simulink model "CRIT4INDIFullLoop"  (R2019b)
settings: Solver=VariableStepAuto  StartTime=0.0  StopTime=50  RelTol=1e-3
values from neighbouring files (symbols this model uses):
  Ahg2 = blkdiag(Ahg2, Ahcg)    [HinFSynINDIFullLoop.m]
  Ahs3 = blkdiag(Ahs3, Ahcs)    [HinFSynINDIFullLoop.m]
  Ahs7 = blkdiag(Ahs7, Ahcs)    [HinFSynINDIFullLoop.m]
  Amc = d2c(Amd,'tustin')    [HinFSynINDIFullLoop.m]
  Asc = d2c(Asd,'tustin')    [HinFSynINDIFullLoop.m]
  Bhg2 = blkdiag(Bhg2, Bhcg)    [HinFSynINDIFullLoop.m]
  Bhs3 = blkdiag(Bhs3, Bhcs)    [HinFSynINDIFullLoop.m]
  Bhs7 = blkdiag(Bhs7, Bhcs)    [HinFSynINDIFullLoop.m]
  Chg2 = blkdiag(Chg2, Chcg)    [HinFSynINDIFullLoop.m]
  Chs3 = blkdiag(Chs3, Chcs)    [HinFSynINDIFullLoop.m]
  Chs7 = blkdiag(Chs7, Chcs)    [HinFSynINDIFullLoop.m]
  Dhg2 = blkdiag(Dhg2, Dhcg)    [HinFSynINDIFullLoop.m]
  Dhs3 = blkdiag(Dhs3, Dhcs)    [HinFSynINDIFullLoop.m]
  Dhs7 = blkdiag(Dhs7, Dhcs)    [HinFSynINDIFullLoop.m]
  Gs = [-10.67  10.67  0     0     0     0 0 ... (first row only)    [HinFSynINDIFullLoop.m]
  Gs_inv = pinv(Gs)    [HinFSynINDIFullLoop.m]
  Gs_thrust = [0 0 0 0 0 0 0 ... (first row only)    [HinFSynINDIFullLoop.m]
  Kdg = diag([2.0; 1.8])    [HinFSynINDIFullLoop.m]
  Kds = [10; 18; 18]    [HinFSynINDIFullLoop.m]
  Kpg = blkdiag(Kposx.D,Kposz.D)    [HinFSynINDIFullLoop.m]
  Kps = [4.1089; 4.7304; 7.36]    [HinFSynINDIFullLoop.m]
settings Model: Creator=AutomZ2-RG02A02  LastModifiedBy=demouran
settings DebuggingCC: SFMachineParentedDataDiag=error

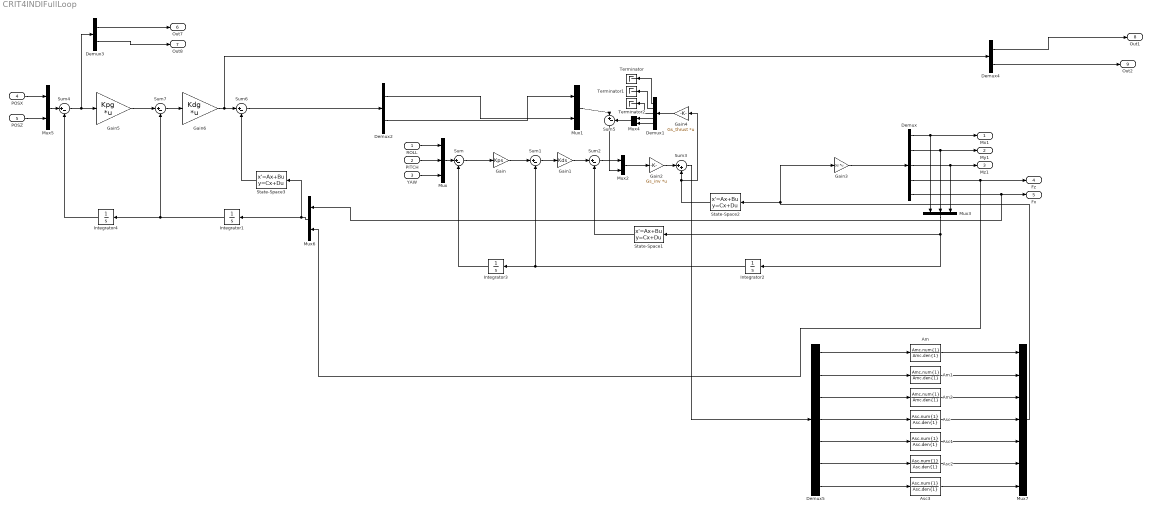
== system CRIT4INDIFullLoop ==
  ROLL : Inport
  PITCH : Inport  Port=2
  YAW : Inport  Port=3
  POSX : Inport  Port=4
  POSZ : Inport  Port=5
  Am : TransferFcn  Numerator=Amc.num{1}  Denominator=Amc.den{1}
  Am1 : TransferFcn  Numerator=Amc.num{1}  Denominator=Amc.den{1}
  Am2 : TransferFcn  Numerator=Amc.num{1}  Denominator=Amc.den{1}
  Asc{,1..3} (4 alike) : TransferFcn  Numerator=Asc.num{1}  Denominator=Asc.den{1}
  Demux : Demux  Outputs=5
  Demux1 : Demux  Outputs=5
  Demux2 : Demux  Outputs=2
  Demux3 : Demux  Outputs=2
  Demux4 : Demux  Outputs=2
  Demux5 : Demux  Outputs=7
  Gain : Gain  Gain=Kps
  Gain1 : Gain  Gain=Kds
  Gain2 : Gain  Gain=Gs_inv  Multiplication=Matrix(K*u)
  Gain3 : Gain  Gain=Gs  Multiplication=Matrix(K*u)
  Gain4 : Gain  Gain=Gs_thrust  Multiplication=Matrix(K*u)
  Gain5 : Gain  Gain=Kpg  Multiplication=Matrix(K*u)
  Gain6 : Gain  Gain=Kdg  Multiplication=Matrix(K*u)
  Integrator{1..4} (4 alike) : Integrator
  Mux : Mux  Inputs=3
  Mux{1,4..6} (4 alike) : Mux  Inputs=2
  Mux2 : Mux  Inputs=[3 2]
  Mux3 : Mux  Inputs=3
  Mux7 : Mux  Inputs=7
  State-Space1 : StateSpace  A=Ahs3  B=Bhs3  C=Chs3  D=Dhs3  InitialCondition=0
  State-Space2 : StateSpace  A=Ahs7  B=Bhs7  C=Chs7  D=Dhs7  InitialCondition=0
  State-Space3 : StateSpace  A=Ahg2  B=Bhg2  C=Chg2  D=Dhg2  InitialCondition=0
  Sum{,1..2,4..7} (7 alike) : Sum  Inputs=|+-
  Sum3 : Sum  Inputs=|++
  Terminator : Terminator
  Terminator1 : Terminator
  Terminator2 : Terminator
  Mx1 : Outport
  My1 : Outport  Port=2
  Mz1 : Outport  Port=3
  Fz : Outport  Port=4
  Fx : Outport  Port=5
  Out7 : Outport  Port=6
  Out8 : Outport  Port=7
  Out1 : Outport  Port=8
  Out2 : Outport  Port=9
  wires:
  Demux1/3 -> Terminator2/1
  State-Space1/1 -> Sum2/2
  Mux4/1 -> Sum5/2
  Mux7/1 -> Gain3/1, State-Space2/1
  Mux/1 -> Sum/1
  Gain4/1 -> Demux1/1
  Mux3/1 -> State-Space1/1, Integrator2/1
  Sum1/1 -> Gain1/1
  State-Space2/1 -> Gain4/1, Sum3/2
  Integrator2/1 -> Sum1/2, Integrator3/1
  Sum2/1 -> Mux2/1
  Sum5/1 -> Mux2/2
  ROLL/1 -> Mux/1
  Demux1/4 -> Mux4/1
  Demux1/5 -> Mux4/2
  Demux1/1 -> Terminator/1
  Demux1/2 -> Terminator1/1
  Gain2/1 -> Sum3/1
  Demux/2 -> Mux3/2, My1/1
  Demux/3 -> Mz1/1, Mux3/3
  Gain/1 -> Sum1/1
  Mux2/1 -> Gain2/1
  PITCH/1 -> Mux/2
  Demux/1 -> Mux3/1, Mx1/1
  YAW/1 -> Mux/3
  Mux1/1 -> Sum5/1
  Sum/1 -> Gain/1
  Integrator3/1 -> Sum/2
  Gain1/1 -> Sum2/1
  Gain3/1 -> Demux/1
  Mux6/1 -> Integrator1/1, State-Space3/1
  Integrator1/1 -> Integrator4/1, Sum7/2
  Demux/5 -> Mux6/1, Fx/1
  Sum7/1 -> Gain6/1
  POSX/1 -> Mux5/1
  Gain6/1 -> Demux4/1, Sum6/1
  Demux/4 -> Mux6/2, Fz/1
  Mux5/1 -> Sum4/1
  Gain5/1 -> Sum7/1
  Integrator4/1 -> Sum4/2
  Sum6/1 -> Demux2/1
  State-Space3/1 -> Sum6/2
  POSZ/1 -> Mux5/2
  Demux3/2 -> Out8/1
  Sum4/1 -> Gain5/1, Demux3/1
  Demux3/1 -> Out7/1
  Demux4/2 -> Out2/1
  Demux4/1 -> Out1/1
  Demux5/6 -> Asc2/1
  Demux5/1 -> Am/1
  Am2/1 -> Mux7/3
  Sum3/1 -> Demux5/1
  Asc3/1 -> Mux7/7
  Asc2/1 -> Mux7/6
  Am/1 -> Mux7/1
  Am1/1 -> Mux7/2
  Demux5/5 -> Asc1/1
  Demux5/7 -> Asc3/1
  Asc/1 -> Mux7/4
  Demux5/2 -> Am1/1
  Demux5/4 -> Asc/1
  Demux5/3 -> Am2/1
  Asc1/1 -> Mux7/5
  Demux2/1 -> Mux1/2
  Demux2/2 -> Mux1/1
